simulink model "UR5Model"  (Simulink 8.3)
settings: Solver=ode1  StartTime=0.0  StopTime=tf  FixedStep=Ts  RelTol=1e-3
values from neighbouring files (symbols this model uses):
  qi = [0;0;0;0;0;0]    [initial.m]
settings Model: Creator=H3  LastModifiedBy=H3
settings DataIOCC: SignalLoggingSaveFormat=Dataset
settings DebuggingCC: UnderspecifiedInitializationDetection=Simplified  StateNameClashWarn=none
settings GRTTargetCC: CombineOutputUpdateFcns=on  GRTInterface=off

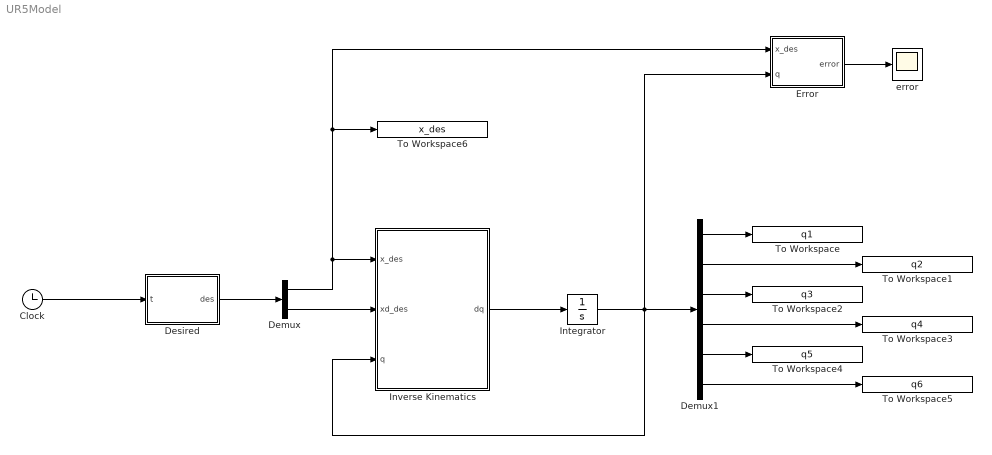
== system UR5Model ==
  Clock : Clock
  Demux : Demux  Outputs=2
  Demux1 : Demux  Outputs=6
  Desired : MATLAB Function  TreatAsAtomicUnit=on
  Error : MATLAB Function  TreatAsAtomicUnit=on
  Integrator : Integrator  InitialCondition=qi
  Inverse Kinematics : MATLAB Function  TreatAsAtomicUnit=on
  To Workspace : ToWorkspace  VariableName=q1  SampleTime=-1
  To Workspace1 : ToWorkspace  VariableName=q2  SampleTime=-1
  To Workspace2 : ToWorkspace  VariableName=q3  SampleTime=-1
  To Workspace3 : ToWorkspace  VariableName=q4  SampleTime=-1
  To Workspace4 : ToWorkspace  VariableName=q5  SampleTime=-1
  To Workspace5 : ToWorkspace  VariableName=q6  SampleTime=-1
  To Workspace6 : ToWorkspace  VariableName=x_des  SampleTime=-1
  error : Scope
  wires:
  Clock/1 -> Desired/1(t)
  Desired/1(des) -> Demux/1
  Demux/1 -> Error/1(x_des), To Workspace6/1, Inverse Kinematics/1(x_des)
  Demux/2 -> Inverse Kinematics/2(xd_des)
  Inverse Kinematics/1(dq) -> Integrator/1
  Integrator/1 -> Error/2(q), Demux1/1, Inverse Kinematics/3(q)
  Demux1/1 -> To Workspace/1
  Demux1/2 -> To Workspace1/1
  Demux1/3 -> To Workspace2/1
  Demux1/4 -> To Workspace3/1
  Demux1/5 -> To Workspace4/1
  Demux1/6 -> To Workspace5/1
  Error/1(error) -> error/1

== matlab function Inverse Kinematics ==
  data: x_des input double; dq output double; xd_des input double; q input double
function dq = IK(x_des,xd_des,q)

q1 = q(1);
q2 = q(2);
q3 = q(3);
q4 = q(4);
q5 = q(5);
q6 = q(6);

%%
x = [(379*cos(q2 + q3)*cos(q1)*sin(q4))/4 - 425*cos(q1)*cos(q2) - (165*cos(q5)*sin(q1))/2 - (165*cos(q2 + q3 + q4)*cos(q1)*sin(q5))/2 - (1093*sin(q1))/10 + (379*sin(q2 + q3)*cos(q1)*cos(q4))/4 - 392*cos(q1)*cos(q2)*cos(q3) + 392*cos(q1)*sin(q2)*sin(q3);
(1093*cos(q1))/10 + (165*cos(q1)*cos(q5))/2 - 425*cos(q2)*sin(q1) + 392*sin(q1)*sin(q2)*sin(q3) - (165*cos(q2 + q3 + q4)*sin(q1)*sin(q5))/2 + (379*cos(q2 + q3)*sin(q1)*sin(q4))/4 + (379*sin(q2 + q3)*cos(q4)*sin(q1))/4 - 392*cos(q2)*cos(q3)*sin(q1);
392*sin(q2 + q3) + 425*sin(q2) + sin(q5)*((165*cos(q2 + q3)*sin(q4))/2 + (165*sin(q2 + q3)*cos(q4))/2) + (379*cos(q2 + q3)*cos(q4))/4 - (379*sin(q2 + q3)*sin(q4))/4 + 446/5;
0;0;0];

%%
J = [ 425*cos(q2)*sin(q1) - (165*cos(q1)*cos(q5))/2 - (1093*cos(q1))/10 - 392*sin(q1)*sin(q2)*sin(q3) + (165*cos(q2 + q3 + q4)*sin(q1)*sin(q5))/2 - (379*cos(q2 + q3)*sin(q1)*sin(q4))/4 - (379*sin(q2 + q3)*cos(q4)*sin(q1))/4 + 392*cos(q2)*cos(q3)*sin(q1), cos(q1)*(392*sin(q2 + q3) + 425*sin(q2) + sin(q5)*((165*cos(q2 + q3)*sin(q4))/2 + (165*sin(q2 + q3)*cos(q4))/2) + (379*cos(q2 + q3)*cos(q4))/4 - (379*sin(q2 + q3)*sin(q4))/4),                     cos(q1)*((379*cos(q2 + q3 + q4))/4 + 392*sin(q2 + q3) + (165*sin(q2 + q3 + q4)*sin(q5))/2),                     cos(q1)*((379*cos(q2 + q3 + q4))/4 + (165*sin(q2 + q3 + q4)*sin(q5))/2), (165*sin(q1)*sin(q5))/2 - (165*cos(q1)*cos(q2)*cos(q3)*cos(q4)*cos(q5))/2 + (165*cos(q1)*cos(q2)*cos(q5)*sin(q3)*sin(q4))/2 + (165*cos(q1)*cos(q3)*cos(q5)*sin(q2)*sin(q4))/2 + (165*cos(q1)*cos(q4)*cos(q5)*sin(q2)*sin(q3))/2,                                                     0;
 (379*cos(q2 + q3)*cos(q1)*sin(q4))/4 - 425*cos(q1)*cos(q2) - (165*cos(q5)*sin(q1))/2 - (165*cos(q2 + q3 + q4)*cos(q1)*sin(q5))/2 - (1093*sin(q1))/10 + (379*sin(q2 + q3)*cos(q1)*cos(q4))/4 - 392*cos(q1)*cos(q2)*cos(q3) + 392*cos(q1)*sin(q2)*sin(q3), sin(q1)*(392*sin(q2 + q3) + 425*sin(q2) + sin(q5)*((165*cos(q2 + q3)*sin(q4))/2 + (165*sin(q2 + q3)*cos(q4))/2) + (379*cos(q2 + q3)*cos(q4))/4 - (379*sin(q2 + q3)*sin(q4))/4),                     sin(q1)*((379*cos(q2 + q3 + q4))/4 + 392*sin(q2 + q3) + (165*sin(q2 + q3 + q4)*sin(q5))/2),                     sin(q1)*((379*cos(q2 + q3 + q4))/4 + (165*sin(q2 + q3 + q4)*sin(q5))/2), (165*cos(q2)*cos(q5)*sin(q1)*sin(q3)*sin(q4))/2 - (165*cos(q2)*cos(q3)*cos(q4)*cos(q5)*sin(q1))/2 - (165*cos(q1)*sin(q5))/2 + (165*cos(q3)*cos(q5)*sin(q1)*sin(q2)*sin(q4))/2 + (165*cos(q4)*cos(q5)*sin(q1)*sin(q2)*sin(q3))/2,                                                     0;
                                                                                                                                                                                                                                                       0,                                                   (165*sin(q2 + q3 + q4 + q5))/4 - (379*sin(q2 + q3 + q4))/4 + 392*cos(q2 + q3) + 425*cos(q2) - (165*sin(q2 + q3 + q4 - q5))/4, (165*sin(q2 + q3 + q4 + q5))/4 - (379*sin(q2 + q3 + q4))/4 + 392*cos(q2 + q3) - (165*sin(q2 + q3 + q4 - q5))/4, (165*sin(q2 + q3 + q4 + q5))/4 - (379*sin(q2 + q3 + q4))/4 - (165*sin(q2 + q3 + q4 - q5))/4,                                                                                                                                                                 (165*sin(q2 + q3 + q4 + q5))/4 + (165*sin(q2 + q3 + q4 - q5))/4,                                                     0;
                                                                                                                                                                                                                                                       0,                                                                                                                                                                       -sin(q1),                                                                                                       -sin(q1),                                                                                    -sin(q1),                                                                                                                                                                                                       sin(q2 + q3 + q4)*cos(q1), - cos(q5)*sin(q1) - cos(q2 + q3 + q4)*cos(q1)*sin(q5);
                                                                                                                                                                                                                                                       0,                                                                                                                                                                        cos(q1),                                                                                                        cos(q1),                                                                                     cos(q1),                                                                                                                                                                                                       sin(q2 + q3 + q4)*sin(q1),   cos(q1)*cos(q5) - cos(q2 + q3 + q4)*sin(q1)*sin(q5);
                                                                                                                                                                                                                                                       1,                                                                                                                                                                              0,                                                                                                              0,                                                                                           0,                                                                                                                                                                                                               cos(q2 + q3 + q4),                             sin(q2 + q3 + q4)*sin(q5)];
%%
k = 1*eye(6);
dq = pinv(J)*(xd_des + k*(x_des-x));

== matlab function Desired ==
  data: t input double; des output double
function des = desired(t)

%% Timing Law
Pi = [-185 -175 900 0 0 0].';
Pf = [-185 -375 636 0 0 0].';
L = norm(Pf(1:3,1)-Pi(1:3,1));

s = 0;
sd = 0;

T = 10;
T_s = T/8;
vmax = L/(T-T_s);
amax = vmax/T_s;

if t<=T_s
    s = amax*t^2/2;
    sd = amax*t;
elseif t>T_s && t<T-T_s
    s = vmax*t - vmax^2/(2*amax);
    sd = vmax;
elseif t>=T-T_s && t<=T
    s = -amax*(t-T)^2/2 + vmax*T - vmax^2/amax;
    sd = vmax - amax*(t-T+T_s);
end

%% Geometric Path
%% Line
Pi = [-185 -175 900 0 0 0].';
Pf = [-185 -375 636 0 0 0].';
L = norm(Pf(1:3,1)-Pi(1:3,1));

x_des = Pi + s*(Pf - Pi)/L;
xd_des = (Pf-Pi)*sd/L;

%% 
des=[x_des;xd_des];

== matlab function Error ==
  data: x_des input double; q input double; error output double
function error = Error(x_des,q)

q1 = q(1);
q2 = q(2);
q3 = q(3);
q4 = q(4);
q5 = q(5);
q6 = q(6);

%%
x = [(379*cos(q2 + q3)*cos(q1)*sin(q4))/4 - 425*cos(q1)*cos(q2) - (165*cos(q5)*sin(q1))/2 - (165*cos(q2 + q3 + q4)*cos(q1)*sin(q5))/2 - (1093*sin(q1))/10 + (379*sin(q2 + q3)*cos(q1)*cos(q4))/4 - 392*cos(q1)*cos(q2)*cos(q3) + 392*cos(q1)*sin(q2)*sin(q3);
(1093*cos(q1))/10 + (165*cos(q1)*cos(q5))/2 - 425*cos(q2)*sin(q1) + 392*sin(q1)*sin(q2)*sin(q3) - (165*cos(q2 + q3 + q4)*sin(q1)*sin(q5))/2 + (379*cos(q2 + q3)*sin(q1)*sin(q4))/4 + (379*sin(q2 + q3)*cos(q4)*sin(q1))/4 - 392*cos(q2)*cos(q3)*sin(q1);
392*sin(q2 + q3) + 425*sin(q2) + sin(q5)*((165*cos(q2 + q3)*sin(q4))/2 + (165*sin(q2 + q3)*cos(q4))/2) + (379*cos(q2 + q3)*cos(q4))/4 - (379*sin(q2 + q3)*sin(q4))/4 + 446/5;
0;0;0];

%%
e = x_des(1:3) - x(1:3);
error = norm(e);
